simulink model "H8_HEMS_partelinealizada"  (R2022b)
settings: Solver=VariableStepAuto  StartTime=0.0  StopTime=10.0  RelTol=1e-3
InitFcn:
  | m = 200;
  | g = 9.81;
  | x_lev12 = 0.443;
  | x_lev34 = 0.542;
  | x_guid12 = 0.4475;
  | x_guid34 = 0.5465;
  | x_lim = 0.0495;
  | y_lev13 = 0.23686;
  | y_lev24 = 0.23686;
  | y_guid13 = 0.24263;
  | y_guid24 = 0.24263;
  | y_lim = 0.0005;
  | y_brk = 0.21552;
  | z_lev = 0.08546;
  | z_guid = 0.026;
  | z_lim = 0.1055;
  | z_brk = 0.03941;
  | kp_lev = 50;
  | ki_lev = 400;
  | kp_guid = 6;
  | ki_guid = 46.5;
  | Imax_lev = 50;
  | Imin_lev = -50;
  | Imax_guid = 50;
  | Imin_guid = 0;
  | cg_nom = 0.567;
  | I = [43.082 0 0; 0 26.887 0; 0 0 29.297]
values from neighbouring files (symbols this model uses):
  cg_suelo = 0.56985    [linealizacion_HEMS.m]
  cg_techo = 0.55735    [linealizacion_HEMS.m]
undefined symbols (not defined in the file or in its folder): hems
libraries: shared6dof x1
settings Model: Creator=USUARIO  LastModifiedBy=aceao

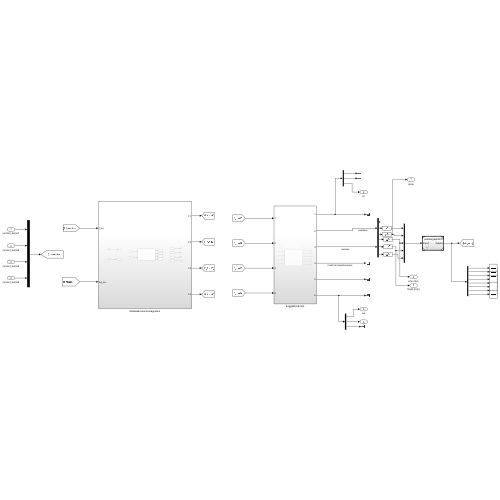
[thumbnail: Simulink's stored preview of the top-level diagram]
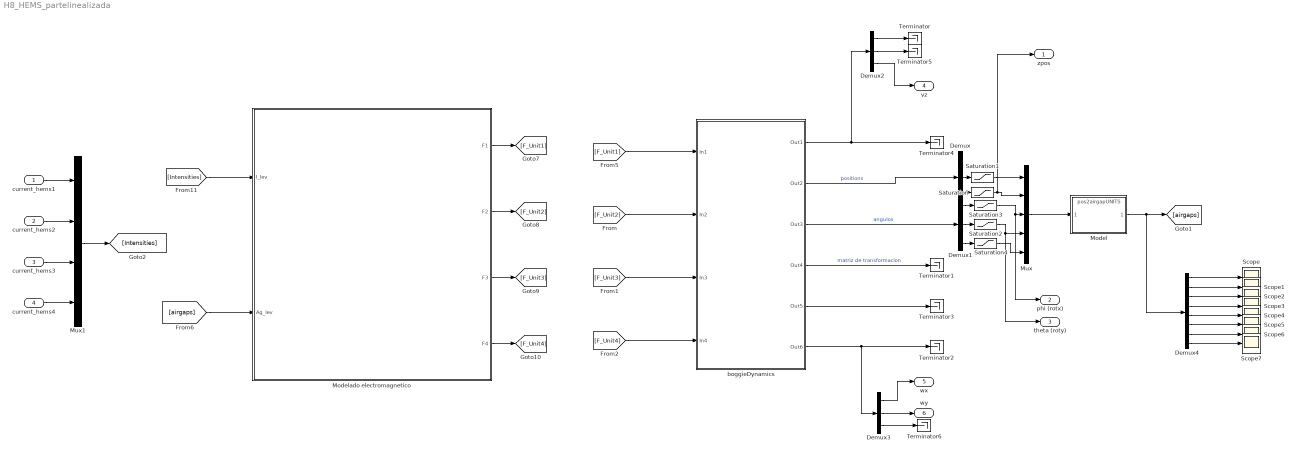
== system H8_HEMS_partelinealizada ==
  current_hems1 : Inport
  current_hems2 : Inport  Port=2
  current_hems3 : Inport  Port=3
  current_hems4 : Inport  Port=4
  Demux{,1..3} (4 alike) : Demux  Outputs=3
  Demux4 : Demux  Outputs=8
  Model : ModelReference  ModelNameDialog=pos2airgapUNITS.slx  SimulationMode=Normal  ModelReferenceVersion=1.3
  Modelado electromagnetico : Subsystem
  Mux : Mux  Inputs=5
  Mux1 : Mux
  Saturation : Saturate  UpperLimit=cg_suelo  LowerLimit=cg_techo
  Saturation1 : Saturate  UpperLimit=0.012  LowerLimit=-0.012
  Saturation2 : Saturate  UpperLimit=0.01268  LowerLimit=-0.01268
  Saturation3 : Saturate  UpperLimit=0.0476  LowerLimit=-0.0476
  Saturation4 : Saturate  UpperLimit=0.024  LowerLimit=-0.024
  Scope{,1..7} (8 alike) : Scope
  Terminator{,1..6} (7 alike) : Terminator
  boggieDynamics : Subsystem
  zpos : Outport
  phi (rotx) : Outport  Port=2
  theta (roty) : Outport  Port=3
  vz : Outport  Port=4
  wx : Outport  Port=5
  wy : Outport  Port=6
  wires:
  boggieDynamics/3(Out3) -> Demux1/1  "angulos"
  boggieDynamics/6(Out6) -> Terminator2/1, Demux3/1
  Saturation1/1 -> Mux/1
  Demux1/2 -> Saturation2/1
  Demux4/1 -> Scope/1
  boggieDynamics/4(Out4) -> Terminator1/1  "matriz de transformacion"
  Demux4/7 -> Scope6/1
  Saturation/1 -> zpos/1, Mux/2
  [Intensities] -> Modelado electromagnetico/1(I_lev)
  Demux/3 -> Saturation/1
  [F_Unit3] -> boggieDynamics/3(In3)
  Demux/2 -> Saturation1/1
  [F_Unit4] -> boggieDynamics/4(In4)
  Demux4/4 -> Scope3/1
  current_hems2/1 -> Mux1/2
  Model/1 -> Demux4/1, [airgaps]
  Demux4/3 -> Scope2/1
  Demux4/6 -> Scope5/1
  Demux3/2 -> wy/1
  Saturation4/1 -> Mux/5
  Mux/1 -> Model/1
  Saturation2/1 -> theta (roty)/1, Mux/4
  Modelado electromagnetico/1(F1) -> [F_Unit1]
  Demux4/8 -> Scope7/1
  [airgaps] -> Modelado electromagnetico/2(Ag_lev)
  Modelado electromagnetico/4(F4) -> [F_Unit4]
  Demux4/2 -> Scope1/1
  Demux4/5 -> Scope4/1
  Demux2/3 -> vz/1
  Demux3/1 -> wx/1
  Demux1/1 -> Saturation3/1
  Demux1/3 -> Saturation4/1
  Saturation3/1 -> phi (rotx)/1, Mux/3
  [F_Unit1] -> boggieDynamics/1(In1)
  Modelado electromagnetico/3(F3) -> [F_Unit3]
  [F_Unit2] -> boggieDynamics/2(In2)
  boggieDynamics/1(Out1) -> Terminator4/1, Demux2/1
  current_hems3/1 -> Mux1/3
  current_hems4/1 -> Mux1/4
  boggieDynamics/2(Out2) -> Demux/1  "positions"
  Mux1/1 -> [Intensities]
  boggieDynamics/5(Out5) -> Terminator3/1
  Modelado electromagnetico/2(F2) -> [F_Unit2]
  current_hems1/1 -> Mux1/1
  Demux2/1 -> Terminator/1
  Demux2/2 -> Terminator5/1
  Demux3/3 -> Terminator6/1

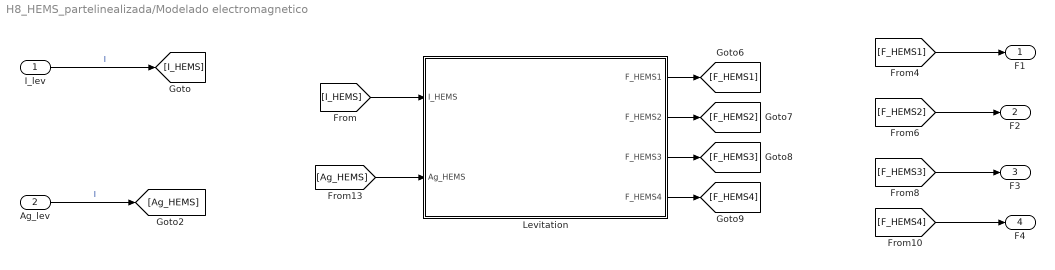
== system H8_HEMS_partelinealizada/Modelado electromagnetico ==
  I_lev : Inport
  Ag_lev : Inport  Port=2
  Levitation : Subsystem
  F1 : Outport
  F2 : Outport  Port=2
  F3 : Outport  Port=3
  F4 : Outport  Port=4
  wires:
  I_lev/1 -> [I_HEMS]  "I"
  [I_HEMS] -> Levitation/1(I_HEMS)
  Levitation/1(F_HEMS1) -> [F_HEMS1]
  Levitation/2(F_HEMS2) -> [F_HEMS2]
  Levitation/3(F_HEMS3) -> [F_HEMS3]
  Levitation/4(F_HEMS4) -> [F_HEMS4]
  [F_HEMS1] -> F1/1
  [F_HEMS2] -> F2/1
  [F_HEMS3] -> F3/1
  [F_HEMS4] -> F4/1
  [Ag_HEMS] -> Levitation/2(Ag_HEMS)
  Ag_lev/1 -> [Ag_HEMS]  "I"

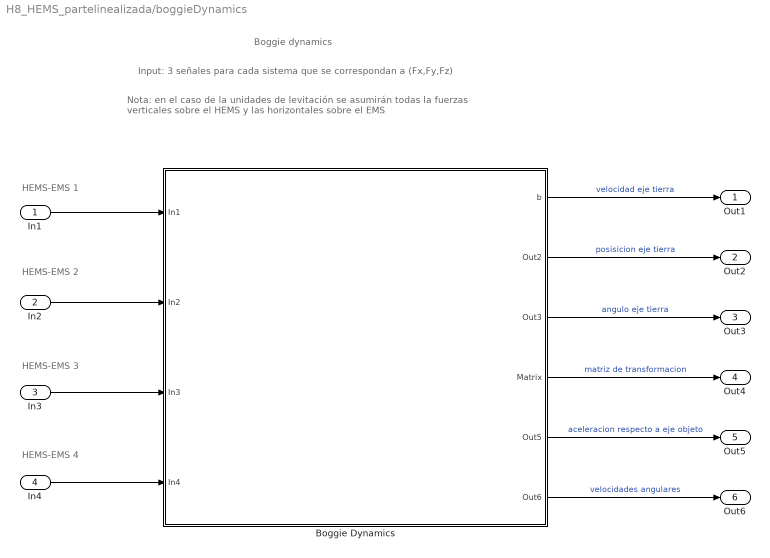
== system H8_HEMS_partelinealizada/boggieDynamics ==
  note: Input: 3 señales para cada sistema que se correspondan a (Fx,Fy,Fz)
  note: HEMS-EMS 3
  note: HEMS-EMS 1
  note: HEMS-EMS 4
  note: HEMS-EMS 2
  note: Boggie dynamics
  note: Nota: en el caso de la unidades de levitación se asumirán todas la fuerzas
      | verticales sobre el HEMS y las horizontales sobre el EMS
  In1 : Inport
  In2 : Inport  Port=2
  In3 : Inport  Port=3
  In4 : Inport  Port=4
  Boggie Dynamics : Subsystem
      mask Display: image('C:\UPV\Hyperloop\Levitacion\ejes.png'); % Use "Edit Image" on toolstrip to change.
  Out1 : Outport
  Out2 : Outport  Port=2
  Out3 : Outport  Port=3
  Out4 : Outport  Port=4
  Out5 : Outport  Port=5
  Out6 : Outport  Port=6
  wires:
  Boggie Dynamics/4(Matrix) -> Out4/1  "matriz de transformacion"
  Boggie Dynamics/6(Out6) -> Out6/1  "velocidades angulares"
  Boggie Dynamics/5(Out5) -> Out5/1  "aceleracion respecto a eje objeto"
  In1/1 -> Boggie Dynamics/1(In1)
  In3/1 -> Boggie Dynamics/3(In3)
  In4/1 -> Boggie Dynamics/4(In4)
  Boggie Dynamics/1(b) -> Out1/1  "velocidad eje tierra"
  In2/1 -> Boggie Dynamics/2(In2)
  Boggie Dynamics/2(Out2) -> Out2/1  "posisicion eje tierra"
  Boggie Dynamics/3(Out3) -> Out3/1  "angulo eje tierra"

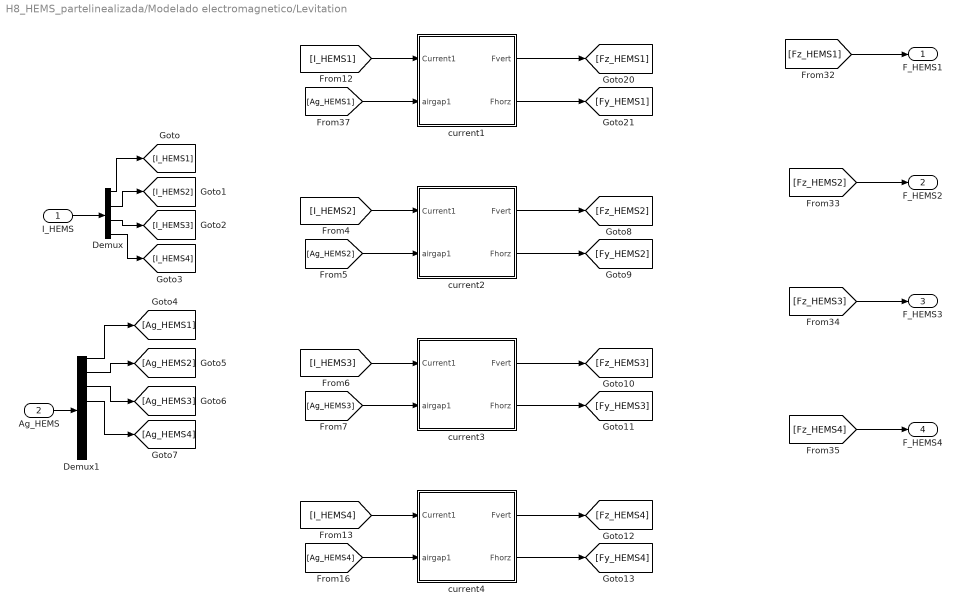
== system H8_HEMS_partelinealizada/Modelado electromagnetico/Levitation ==
  I_HEMS : Inport
  Ag_HEMS : Inport  Port=2
  Demux : Demux
  Demux1 : Demux  Outputs=8
  current1 : Subsystem
  current2 : Subsystem
  current3 : Subsystem
  current4 : Subsystem
  F_HEMS1 : Outport
  F_HEMS2 : Outport  Port=2
  F_HEMS3 : Outport  Port=3
  F_HEMS4 : Outport  Port=4
  wires:
  I_HEMS/1 -> Demux/1
  Demux/1 -> [I_HEMS1]
  Demux/2 -> [I_HEMS2]
  Demux/3 -> [I_HEMS3]
  Demux/4 -> [I_HEMS4]
  Demux1/2 -> [Ag_HEMS2]
  Demux1/3 -> [Ag_HEMS3]
  Ag_HEMS/1 -> Demux1/1
  Demux1/4 -> [Ag_HEMS4]
  Demux1/1 -> [Ag_HEMS1]
  [Fz_HEMS1] -> F_HEMS1/1
  [Fz_HEMS2] -> F_HEMS2/1
  [Fz_HEMS3] -> F_HEMS3/1
  [Fz_HEMS4] -> F_HEMS4/1
  current1/1(Fvert) -> [Fz_HEMS1]
  current1/2(Fhorz) -> [Fy_HEMS1]
  [I_HEMS1] -> current1/1(Current1)
  [Ag_HEMS1] -> current1/2(airgap1)
  current2/1(Fvert) -> [Fz_HEMS2]
  [Ag_HEMS2] -> current2/2(airgap1)
  current2/2(Fhorz) -> [Fy_HEMS2]
  [I_HEMS2] -> current2/1(Current1)
  current3/1(Fvert) -> [Fz_HEMS3]
  [Ag_HEMS3] -> current3/2(airgap1)
  [I_HEMS4] -> current4/1(Current1)
  [I_HEMS3] -> current3/1(Current1)
  current4/2(Fhorz) -> [Fy_HEMS4]
  current3/2(Fhorz) -> [Fy_HEMS3]
  current4/1(Fvert) -> [Fz_HEMS4]
  [Ag_HEMS4] -> current4/2(airgap1)

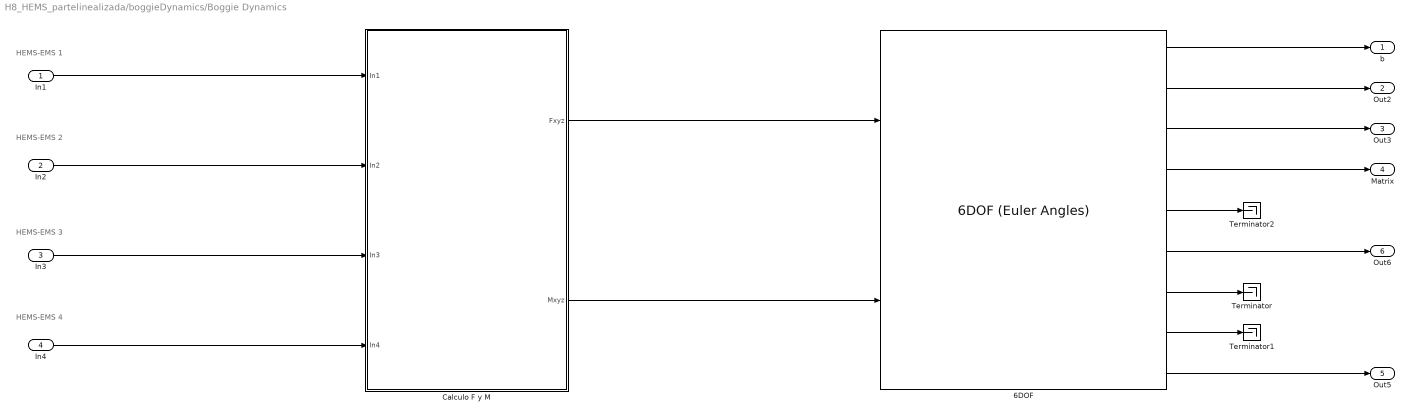
== system H8_HEMS_partelinealizada/boggieDynamics/Boggie Dynamics ==
  note: HEMS-EMS 1
  note: HEMS-EMS 2
  note: HEMS-EMS 3
  note: HEMS-EMS 4
  In1 : Inport
  In2 : Inport  Port=2
  In3 : Inport  Port=3
  In4 : Inport  Port=4
  "6DOF " : shared6dof/6DOF (Euler Angles)  units=Metric (MKS)  mtype=Fixed  rep=Euler Angles  xme_0=[0 0 cg_nom]  Vm_0=[0 0 0]  eul_0=[0 0 0]  pm_0=[0 0 0]  mass_0=m  mass_e=0.5  mass_f=2.0  inertia=I  inertia_e=eye(3)  inertia_f=2*eye(3)  k_quat=1.0  vre_flag=on  abi_flag=on  aMode=0  xme_statename=''  Vm_statename=''  eul_statename=''  quat_statename=''  pm_statename=''  mass_statename=''
  Calculo F y M : Subsystem
  Terminator : Terminator
  Terminator1 : Terminator
  Terminator2 : Terminator
  b : Outport
  Out2 : Outport  Port=2
  Out3 : Outport  Port=3
  Matrix : Outport  Port=4
  Out5 : Outport  Port=5
  Out6 : Outport  Port=6
  wires:
  "6DOF "/1 -> b/1
  "6DOF "/2 -> Out2/1
  "6DOF "/3 -> Out3/1
  In1/1 -> Calculo F y M/1(In1)
  In2/1 -> Calculo F y M/2(In2)
  In3/1 -> Calculo F y M/3(In3)
  In4/1 -> Calculo F y M/4(In4)
  "6DOF "/6 -> Out6/1
  "6DOF "/8 -> Terminator1/1
  "6DOF "/7 -> Terminator/1
  Calculo F y M/1(Fxyz) -> "6DOF "/1
  Calculo F y M/2(Mxyz) -> "6DOF "/2
  "6DOF "/4 -> Matrix/1
  "6DOF "/9 -> Out5/1
  "6DOF "/5 -> Terminator2/1

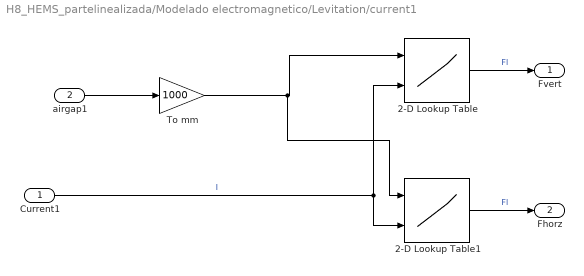
== system H8_HEMS_partelinealizada/Modelado electromagnetico/Levitation/current1 ==
  Current1 : Inport
  airgap1 : Inport  Port=2
  2-D Lookup Table : Lookup_n-D  BreakpointsForDimension1=hems.Airgap'  BreakpointsForDimension2=hems.Current  Table=hems.Force_Vertical  InternalRulePriority=Speed  RndMeth=Simplest
      settings: InputPortMap=u0,u1
  2-D Lookup Table1 : Lookup_n-D  BreakpointsForDimension1=hems.Airgap'  BreakpointsForDimension2=hems.Current  Table=hems.Force_Horizontal  InternalRulePriority=Speed  RndMeth=Simplest
      settings: InputPortMap=u0,u1
  To mm : Gain  Gain=1000
  Fvert : Outport
  Fhorz : Outport  Port=2
  wires:
  2-D Lookup Table1/1 -> Fhorz/1  "Fl"
  2-D Lookup Table/1 -> Fvert/1  "Fl"
  Current1/1 -> 2-D Lookup Table1/2, 2-D Lookup Table/2  "I"
  airgap1/1 -> To mm/1
  To mm/1 -> 2-D Lookup Table1/1, 2-D Lookup Table/1

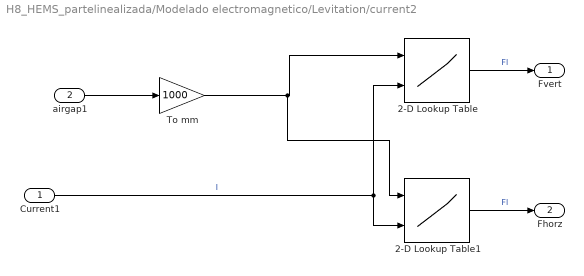
== system H8_HEMS_partelinealizada/Modelado electromagnetico/Levitation/current2 ==
  Current1 : Inport
  airgap1 : Inport  Port=2
  2-D Lookup Table : Lookup_n-D  BreakpointsForDimension1=hems.Airgap'  BreakpointsForDimension2=hems.Current  Table=hems.Force_Vertical  InternalRulePriority=Speed  RndMeth=Simplest
      settings: InputPortMap=u0,u1
  2-D Lookup Table1 : Lookup_n-D  BreakpointsForDimension1=hems.Airgap'  BreakpointsForDimension2=hems.Current  Table=hems.Force_Horizontal  InternalRulePriority=Speed  RndMeth=Simplest
      settings: InputPortMap=u0,u1
  To mm : Gain  Gain=1000
  Fvert : Outport
  Fhorz : Outport  Port=2
  wires:
  2-D Lookup Table1/1 -> Fhorz/1  "Fl"
  2-D Lookup Table/1 -> Fvert/1  "Fl"
  Current1/1 -> 2-D Lookup Table1/2, 2-D Lookup Table/2  "I"
  airgap1/1 -> To mm/1
  To mm/1 -> 2-D Lookup Table1/1, 2-D Lookup Table/1

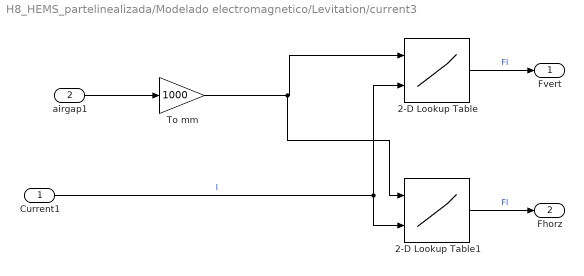
== system H8_HEMS_partelinealizada/Modelado electromagnetico/Levitation/current3 ==
  Current1 : Inport
  airgap1 : Inport  Port=2
  2-D Lookup Table : Lookup_n-D  BreakpointsForDimension1=hems.Airgap'  BreakpointsForDimension2=hems.Current  Table=hems.Force_Vertical  InternalRulePriority=Speed  RndMeth=Simplest
      settings: InputPortMap=u0,u1
  2-D Lookup Table1 : Lookup_n-D  BreakpointsForDimension1=hems.Airgap'  BreakpointsForDimension2=hems.Current  Table=hems.Force_Horizontal  InternalRulePriority=Speed  RndMeth=Simplest
      settings: InputPortMap=u0,u1
  To mm : Gain  Gain=1000
  Fvert : Outport
  Fhorz : Outport  Port=2
  wires:
  2-D Lookup Table1/1 -> Fhorz/1  "Fl"
  2-D Lookup Table/1 -> Fvert/1  "Fl"
  Current1/1 -> 2-D Lookup Table1/2, 2-D Lookup Table/2  "I"
  airgap1/1 -> To mm/1
  To mm/1 -> 2-D Lookup Table1/1, 2-D Lookup Table/1

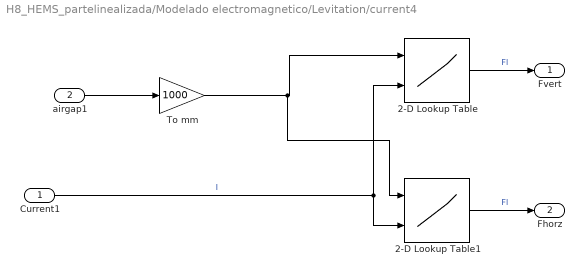
== system H8_HEMS_partelinealizada/Modelado electromagnetico/Levitation/current4 ==
  Current1 : Inport
  airgap1 : Inport  Port=2
  2-D Lookup Table : Lookup_n-D  BreakpointsForDimension1=hems.Airgap'  BreakpointsForDimension2=hems.Current  Table=hems.Force_Vertical  InternalRulePriority=Speed  RndMeth=Simplest
      settings: InputPortMap=u0,u1
  2-D Lookup Table1 : Lookup_n-D  BreakpointsForDimension1=hems.Airgap'  BreakpointsForDimension2=hems.Current  Table=hems.Force_Horizontal  InternalRulePriority=Speed  RndMeth=Simplest
      settings: InputPortMap=u0,u1
  To mm : Gain  Gain=1000
  Fvert : Outport
  Fhorz : Outport  Port=2
  wires:
  2-D Lookup Table1/1 -> Fhorz/1  "Fl"
  2-D Lookup Table/1 -> Fvert/1  "Fl"
  Current1/1 -> 2-D Lookup Table1/2, 2-D Lookup Table/2  "I"
  airgap1/1 -> To mm/1
  To mm/1 -> 2-D Lookup Table1/1, 2-D Lookup Table/1

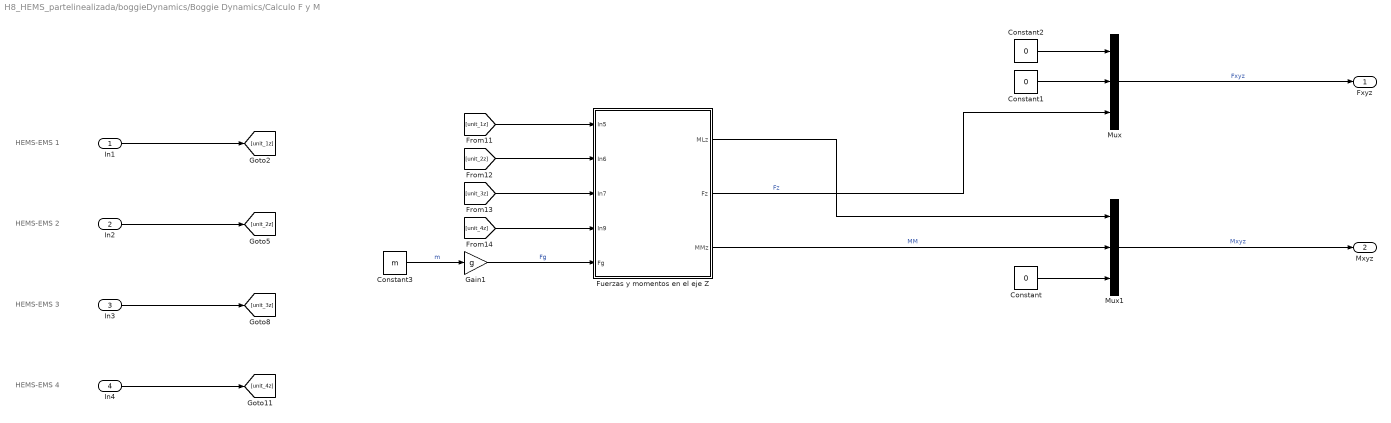
== system H8_HEMS_partelinealizada/boggieDynamics/Boggie Dynamics/Calculo F y M ==
  note: HEMS-EMS 3
  note: HEMS-EMS 1
  note: HEMS-EMS 4
  note: HEMS-EMS 2
  In1 : Inport
  In2 : Inport  Port=2
  In3 : Inport  Port=3
  In4 : Inport  Port=4
  Constant : Constant  Value=0
  Constant1 : Constant  Value=0
  Constant2 : Constant  Value=0
  Constant3 : Constant  Value=m
  Fuerzas y momentos en el eje Z : Subsystem
  Gain1 : Gain  Gain=g
  Mux : Mux  Inputs=3
  Mux1 : Mux  Inputs=3
  Fxyz : Outport
  Mxyz : Outport  Port=2
  wires:
  In3/1 -> [unit_3z]
  Constant3/1 -> Gain1/1  "m"
  Fuerzas y momentos en el eje Z/3(MMz) -> Mux1/2  "MM"
  Mux/1 -> Fxyz/1  "Fxyz"
  Mux1/1 -> Mxyz/1  "Mxyz"
  In1/1 -> [unit_1z]
  Gain1/1 -> Fuerzas y momentos en el eje Z/5(Fg)  "Fg"
  Fuerzas y momentos en el eje Z/2(Fz) -> Mux/3  "Fz"
  Fuerzas y momentos en el eje Z/1(MLz) -> Mux1/1
  In4/1 -> [unit_4z]
  In2/1 -> [unit_2z]
  [unit_1z] -> Fuerzas y momentos en el eje Z/1(In5)
  [unit_3z] -> Fuerzas y momentos en el eje Z/3(In7)
  [unit_2z] -> Fuerzas y momentos en el eje Z/2(In6)
  [unit_4z] -> Fuerzas y momentos en el eje Z/4(In9)
  Constant/1 -> Mux1/3
  Constant1/1 -> Mux/2
  Constant2/1 -> Mux/1

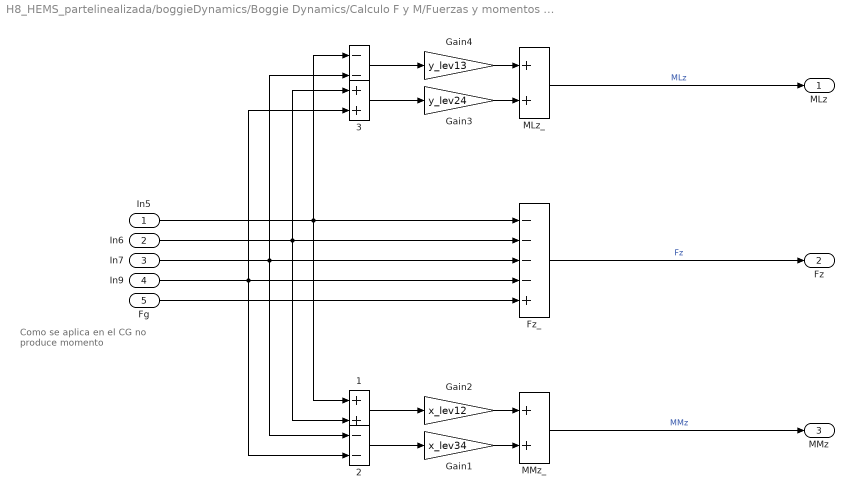
== system H8_HEMS_partelinealizada/boggieDynamics/Boggie Dynamics/Calculo F y M/Fuerzas y momentos en el eje Z ==
  note: Como se aplica en el CG
      |  no produce momento
  In5 : Inport
  In6 : Inport  Port=2
  In7 : Inport  Port=3
  In9 : Inport  Port=4
  Fg : Inport  Port=5
  " " : Sum  Inputs=--
  " 1" : Sum
  " 2" : Sum  Inputs=--
  " 3" : Sum
  " MLz_" : Sum
  " MMz_" : Sum
  Fz_ : Sum  Inputs=----+
  Gain1 : Gain  Gain=x_lev34
  Gain2 : Gain  Gain=x_lev12
  Gain3 : Gain  Gain=y_lev24
  Gain4 : Gain  Gain=y_lev13
  MLz : Outport
  Fz : Outport  Port=2
  MMz : Outport  Port=3
  wires:
  In6/1 -> " 1"/2, Fz_/2, " 3"/1
  " MLz_"/1 -> MLz/1  "MLz"
  Fg/1 -> Fz_/5
  In9/1 -> Fz_/4, " 2"/2, " 3"/2
  In5/1 -> " 1"/1, " "/1, Fz_/1
  In7/1 -> " 2"/1, Fz_/3, " "/2
  Fz_/1 -> Fz/1  "Fz"
  " MMz_"/1 -> MMz/1  "MMz"
  " 3"/1 -> Gain3/1
  " "/1 -> Gain4/1
  Gain4/1 -> " MLz_"/1
  Gain3/1 -> " MLz_"/2
  Gain2/1 -> " MMz_"/1
  " 2"/1 -> Gain1/1
  Gain1/1 -> " MMz_"/2
  " 1"/1 -> Gain2/1
